simulink model "Lab1_LED_FADE_DEMO"  (R2025b)
settings: Solver=FixedStepDiscrete  StartTime=0.0  StopTime=10.0  FixedStep=0.001  RelTol=1e-3  EnableMultiTasking=on
undefined symbols (not defined in the file or in its folder): DiscIntNeverNeededParam, Timer
libraries: MCHP_Blockset x6, simulink x1
(part 2 of 2)

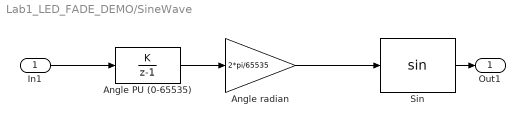
== system Lab1_LED_FADE_DEMO/SineWave ==
  In1 : Inport
  Angle PU (0-65535) : DiscreteIntegrator  IntegratorMethod=Accumulation: Forward Euler  gainval=65535*0.001  SampleTime=.001  OutDataTypeStr=uint16  ICPrevOutput=DiscIntNeverNeededParam  ICPrevScaledInput=DiscIntNeverNeededParam
  Angle radian : Gain  Gain=2*pi/65535  OutDataTypeStr=fixdt(0,16,12)
  Sin : Trigonometry  ApproximationMethod=Lookup
  Out1 : Outport
  wires:
  Angle PU (0-65535)/1 -> Angle radian/1
  Angle radian/1 -> Sin/1
  In1/1 -> Angle PU (0-65535)/1
  Sin/1 -> Out1/1
